simulink model "Tx_BPSK_delta_USRP"  (Simulink 7.4)
settings: Solver=ode45  StartTime=0.0  StopTime=inf  RelTol=1e-3
undefined symbols (not defined in the file): N, S
libraries: dspbuff3 x2, dsparch4 x2, dspsrcs4 x2, commfilt2 x1, usrp_GPP x1
settings Model: Creator=wnieves  LastModifiedBy=bscheers
settings OptimizationCC: InitFltsAndDblsToZero=on

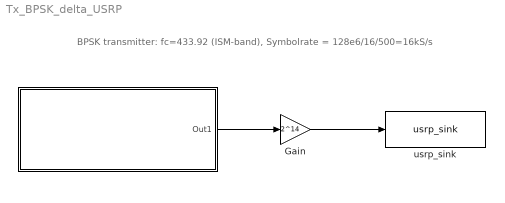
== system Tx_BPSK_delta_USRP ==
  note: BPSK transmitter: fc=433.92 (ISM-band), Symbolrate = 128e6/16/500=16kS/s
  " " : Subsystem  Description=Transmitter
      mask Display: color('red');fprintf('Transmitter')
  Gain : Gain  Gain=2^14  ParameterDataType=sfix(16)  ParameterScaling=2^0  OutDataType=sfix(16)  OutScaling=2^0
  usrp_sink : usrp_GPP/usrp_sink  usrp_number=0  serial_number=S/N: .  decimation=500  sample_width=16 Bit  sampling_rate_and_bandwidth=1 Channels: 256 kSps, 1000 kB/s, 7.8125 Mbit/s.  vector_length=4096  sideA_subdev1_tab_=0  sideA_subdev1_subdevice=Flex 400 Tx MIMO B  sideA_subdev1_datatype=DOUBLE Complex  sideA_subdev1_frequency_range=Min: 400 MHz, Max: 500 MHz.  sideA_subdev1_frequency_port=off  sideA_subdev1_frequency=433.92e6  sideA_subdev1_gain_range=Min: 0 dB, Max: 0 dB, Step Size: 1 dB.  sideA_subdev1_gain=0  sideB_subdev1_tab_=0  sideB_subdev1_subdevice=Flex 400 Tx MIMO B  sideB_subdev1_datatype=Disabled  sideB_subdev1_frequency_range=Min: 400 MHz, Max: 500 MHz.  sideB_subdev1_frequency_port=off  sideB_subdev1_frequency=433.92e6  sideB_subdev1_gain_range=Min: 0 dB, Max: 0 dB, Step Size: 1 dB.  sideB_subdev1_gain=0
  wires:
  ? -> ?
  " "/1(Out1) -> Gain/1
  Gain/1 -> usrp_sink/1

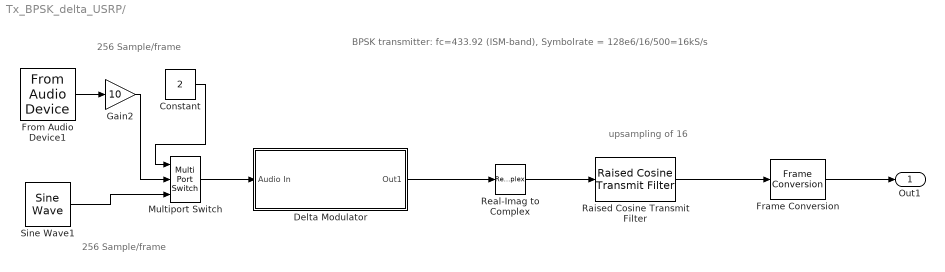
== system Tx_BPSK_delta_USRP/  ==
  note: BPSK transmitter: fc=433.92 (ISM-band), Symbolrate = 128e6/16/500=16kS/s
  note: 256 Sample/frame
  note: upsampling of 16
  note: 256 Sample/frame
  Constant : Constant  Value=2  OutDataType=fixdt(1, 16)  OutScaling=2^0
  Delta Modulator : Subsystem
  Frame Conversion : FrameConversion
  From Audio Device1 : dspsrcs4/From Audio Device  DialogController=dspDDGCreate  DialogControllerArgs=DataTag2  deviceName=Default  numChannels=1  sampleRate=16000  deviceDatatype=Determine from output data type  autoBufferSize=on  bufferSize=4096  queueDuration=1.0  frameSize=256  outputDatatype=single
  Gain2 : Gain  Gain=10  ParameterDataType=fixdt(1, 16)  ParameterScaling=2^0  OutDataType=fixdt(1, 16)  OutScaling=2^0
  Multiport Switch : MultiPortSwitch  Inputs=2  OutDataType=fixdt(1, 16)  OutScaling=2^0
  Raised Cosine Transmit Filter : commfilt2/Raised Cosine Transmit Filter  DialogController=dspDDGCreate  DialogControllerArgs=DataTag3  SystemSampleTime=-1  filtType=Square root  D=8  R=0.35  sampMode=Mute  saveAsFlag=0  framing=Maintain input frame rate  N=16  checkGain=Normalized  filterGain=1  checkCoeff=off  variableName=rcTxFilt  launchFVT=off  roundingMode=Floor  overflowMode=off
  Real-Imag to Complex : RealImagToComplex  Input=Real
  Sine Wave1 : dspsrcs4/Sine Wave  Amplitude=1  Frequency=800  Phase=0  SampleMode=Discrete  OutComplex=Real  CompMethod=Trigonometric fcn  TableSize=Speed  SampleTime=1/16000  SamplesPerFrame=256  dataType=double  wordLen=16  udDataType=sfix(16)  fracBitsMode=Best precision  numFracBits=15  ResetState=Restart at time zero
  Out1 : Outport
  wires:
  Real-Imag to Complex/1 -> Raised Cosine Transmit Filter/1
  Raised Cosine Transmit Filter/1 -> Frame Conversion/1
  Delta Modulator/1(Out1) -> Real-Imag to Complex/1
  Frame Conversion/1 -> Out1/1
  From Audio Device1/1 -> Gain2/1
  Gain2/1 -> Multiport Switch/2
  Sine Wave1/1 -> Multiport Switch/3
  Multiport Switch/1 -> Delta Modulator/1(Audio In)
  Constant/1 -> Multiport Switch/1

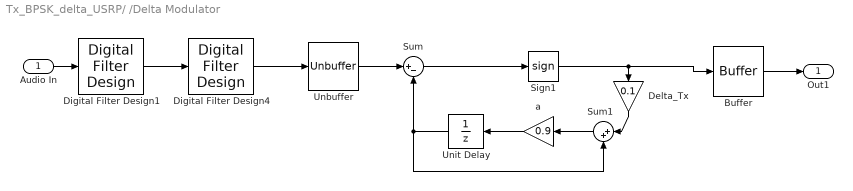
== system Tx_BPSK_delta_USRP/ /Delta Modulator ==
  Audio In : Inport
  Buffer : dspbuff3/Buffer  N=256  V=0  ic=0
  Delta_Tx : Gain  Gain=0.1  ParameterDataType=sfix(16)  ParameterScaling=2^0  OutDataType=sfix(16)  OutScaling=2^0
  Digital Filter Design1 : dsparch4/Digital Filter Design  SystemSampleTime=-1  mwdsp_browser_bugfix_var=off
  Digital Filter Design4 : dsparch4/Digital Filter Design  SystemSampleTime=-1  mwdsp_browser_bugfix_var=off
  Sign1 : Signum
  Sum : Sum  Inputs=|+-  OutDataType=sfix(16)  OutScaling=2^0
  Sum1 : Sum  Inputs=|++  OutDataType=sfix(16)  OutScaling=2^0
  Unbuffer : dspbuff3/Unbuffer  ic=0
  Unit Delay : UnitDelay  SampleTime=-1
  a : Gain  Gain=0.9  ParameterDataType=sfix(16)  ParameterScaling=2^0  OutDataType=sfix(16)  OutScaling=2^0
  Out1 : Outport
  wires:
  Sum/1 -> Sign1/1
  Sign1/1 -> Delta_Tx/1, Buffer/1
  Delta_Tx/1 -> Sum1/1
  Sum1/1 -> a/1
  a/1 -> Unit Delay/1
  Unit Delay/1 -> Sum1/2, Sum/2
  Digital Filter Design1/1 -> Digital Filter Design4/1
  Digital Filter Design4/1 -> Unbuffer/1
  Unbuffer/1 -> Sum/1
  Buffer/1 -> Out1/1
  Audio In/1 -> Digital Filter Design1/1
